simulink library "vhit_control_library"  (R2023a)
settings: Solver=VariableStepAuto  StartTime=0.0  StopTime=10.0  RelTol=1e-3
undefined symbols (not defined in the file): bit, cstElctSpdMaxVal, cstSlowTaskSampTime, parDirCurrMaxVal, parElctSpdMaxVal, parFluxObsFiltCoef, parQdrtCurrMaxVal, parRefSpdFallSlewRate, parRefSpdRisSlewRate, PolePairNum
libraries: lib_conversion x90, lib_square_root x11, lib_dynamic_saturator x9, lib_resettable_unit_delay x2, lib_fault_definiteness x1, lib_angle_mapper x1, lib_cart_to_polar_coor_transformer x1, lib_clarke_transform x1, lib_configurable_parameter x1, lib_current_control_decoupling x1, lib_derating_reference_speed_limiter x1, lib_discrete_time_integrator x1
(part 3 of 3)

== system vhit_control_library/lib_FWReferenceCurrentGenerator_0/vss_ActiveReferenceCurrentStrategy/vss_FieldWeakeningStrategy/sss_CurrentMTPALimitComputation/ias_CurrentMTPALimitAsymmetricMotorCondition ==
  lb_mfPermMagFlux : Inport
  Action Port : ActionPort
  Add1 : Sum  Inputs=+-  OutDataTypeStr=Inherit: Inherit via back propagation
  Add2 : Sum  Inputs=+-  OutDataTypeStr=Inherit: Inherit via back propagation
  Add3 : Sum  OutDataTypeStr=Inherit: Same as first input
  Add4 : Sum  Inputs=+-  OutDataTypeStr=Inherit: Same as first input
  Constant3 : Constant  Value=lb_parQdrtIndc
  Constant4 : Constant  Value=lb_parDirIndc
  Constant5 : Constant  Value=lb_parMaxPhsCurr
  Constant6 : Constant  Value=lb_parMaxPhsCurr
  Data Type Duplicate : DataTypeDuplicate
  Divide1 : Product  Inputs=*/  OutDataTypeStr=Inherit: Inherit via back propagation
  Gain : Gain  Gain=4  OutDataTypeStr=Inherit: Same as input
  Gain1 : Gain  Gain=1/2  OutDataTypeStr=Inherit: Inherit via back propagation
  Square{,1..3} (4 alike) : Math  Operator=square  SignedPower=on  OutDataTypeStr=Inherit: Inherit via back propagation
  lib_SquareRoot_1 : lib_square_root/lib_SquareRoot_0  lb_parLktSize=128  lb_parInpDataType=uint16  lb_parOutpDataType=Inherit: Inherit via back propagation
  lib_SquareRoot_2 : lib_square_root/lib_SquareRoot_0  lb_parLktSize=128  lb_parInpDataType=uint16  lb_parOutpDataType=Inherit: Inherit via back propagation
  lib_s16p29b0_1 : lib_conversion/lib_Conversion_0  lb_parDataType=fixdt(1,16,2^-29,0)  lb_parOutpMaxVal=[]  lb_parOutpMinVal=[]  lb_parSatFlag=off
  lib_s16p7b0_1 : lib_conversion/lib_Conversion_0  lb_parDataType=fixdt(1,16,2^-7,0)  lb_parOutpMaxVal=[]  lb_parOutpMinVal=[]  lb_parSatFlag=off
  lib_u16n0b0_1 : lib_conversion/lib_Conversion_0  lb_parDataType=uint16  lb_parOutpMaxVal=[]  lb_parOutpMinVal=[]  lb_parSatFlag=off
  lib_u16n0b0_2 : lib_conversion/lib_Conversion_0  lb_parDataType=uint16  lb_parOutpMaxVal=[]  lb_parOutpMinVal=[]  lb_parSatFlag=off
  lib_u16n0b0_3 : lib_conversion/lib_Conversion_0  lb_parDataType=uint16  lb_parOutpMaxVal=[]  lb_parOutpMinVal=[]  lb_parSatFlag=off
  lib_u16p2b0_1 : lib_conversion/lib_Conversion_0  lb_parDataType=fixdt(0,16,2^-2,0)  lb_parOutpMaxVal=[]  lb_parOutpMinVal=[]  lb_parSatFlag=off
  lib_u16p4b0_4 : lib_conversion/lib_Conversion_0  lb_parDataType=fixdt(0,16,2^-4,0)  lb_parOutpMaxVal=[]  lb_parOutpMinVal=[]  lb_parSatFlag=off
  lb_iDirCurrMTPALim : Outport
  lb_iQdrtCurrMTPALim : Outport  Port=2
  wires:
  [lb_iDirCurrMTPALim] -> lb_iDirCurrMTPALim/1
  [lb_iQdrtCurrMTPALim] -> lb_iQdrtCurrMTPALim/1
  lb_mfPermMagFlux/1 -> [lb_mfPermMagFlux]
  Square3/1 -> lib_u16n0b0_3/1
  Square2/1 -> lib_u16p4b0_4/1
  lib_u16p4b0_4/1 -> Add4/2
  lib_s16p29b0_1/1 -> Gain/1
  lib_SquareRoot_2/1 -> [lb_iQdrtCurrMTPALim]
  lib_s16p7b0_1/1 -> Data Type Duplicate/1, Add2/1
  Add4/1 -> lib_SquareRoot_2/1
  Divide1/1 -> lib_s16p7b0_1/1, Square/1
  lib_u16p2b0_1/1 -> Add3/2
  Add3/1 -> lib_SquareRoot_1/1
  Constant6/1 -> Square3/1
  Constant5/1 -> Square1/1
  Constant4/1 -> Add1/2
  lib_u16n0b0_3/1 -> Add4/1
  lib_u16n0b0_1/1 -> Add3/1
  [lb_mfPermMagFlux] -> Divide1/1
  Gain1/1 -> lib_u16p2b0_1/1
  Add1/1 -> lib_s16p29b0_1/1
  [lb_iDirCurrMTPALim] -> Square2/1
  Square/1 -> lib_u16n0b0_1/1
  Add2/1 -> [lb_iDirCurrMTPALim]
  Constant3/1 -> Add1/1
  lib_SquareRoot_1/1 -> Data Type Duplicate/2, Add2/2
  lib_u16n0b0_2/1 -> Gain1/1
  Gain/1 -> Divide1/2
  Square1/1 -> lib_u16n0b0_2/1

== system vhit_control_library/lib_FWReferenceCurrentGenerator_0/vss_ActiveReferenceCurrentStrategy/vss_FieldWeakeningStrategy/sss_CurrentMTPALimitComputation/ias_CurrentMTPALimitSymmetricMotorCondition ==
  Action Port : ActionPort
  Constant : Constant  Value=0  OutDataTypeStr=Inherit: Inherit via back propagation
  Constant6 : Constant  Value=lb_parMaxPhsCurr
  Data Type Conversion : DataTypeConversion  SaturateOnIntegerOverflow=off  RndMeth=Floor
  lb_iDirCurrMTPALim : Outport
  lb_iQdrtCurrMTPALim : Outport  Port=2
  wires:
  Data Type Conversion/1 -> lb_iQdrtCurrMTPALim/1
  Constant6/1 -> Data Type Conversion/1
  Constant/1 -> lb_iDirCurrMTPALim/1

== system vhit_control_library/lib_FWReferenceCurrentGenerator_0/vss_ActiveReferenceCurrentStrategy/vss_MaximumTorquePerAmpereStrategy/ias_MTPAControlStrategy/sss_MTPAControlStrategy ==
  lb_tqRefTrq : Inport
  lb_mfPermMagFlux : Inport  Port=2
  Prelookup : PreLookup  BreakpointsData=[10:10:110]  BreakpointsSpecification=Even spacing  BreakpointsNumPoints=lb_parTrqSampNum  BreakpointsFirstPoint=lb_parMTPATrqDataFrstVal  BreakpointsSpacing=lb_parMTPATrqDataStepVal  OutputSelection=Index and fraction as bus  RemoveProtectionInput=on  IndexDataTypeStr=uint16  FractionDataTypeStr=fixdt(0,16,2^-15,0)  RndMeth=Simplest
  Prelookup1 : PreLookup  BreakpointsData=[10:10:110]  BreakpointsSpecification=Even spacing  BreakpointsNumPoints=lb_parTempSampNum  BreakpointsFirstPoint=lb_parMTPAPermMagFluxDataFrstVal  BreakpointsSpacing=lb_parMTPAPermMagFluxDataStepVal  OutputSelection=Index and fraction as bus  RemoveProtectionInput=on  IndexDataTypeStr=uint16  FractionDataTypeStr=fixdt(0,16,2^-15,0)  RndMeth=Simplest
  lib_Conversion_1 : lib_conversion/lib_Conversion_0  lb_parDataType=lb_parOutpDataType  lb_parOutpMaxVal=[]  lb_parOutpMinVal=[]  lb_parSatFlag=off
  lkt_MTPAControlStrategy : Interpolation_n-D  Table=lb_parMTPA2DLktMtrx  ExtrapMethod=Clip  RequireIndexFractionAsBus=on  RemoveProtectionIndex=on  OutDataTypeStr=Inherit: Inherit via back propagation  InternalRulePriority=Speed  RndMeth=Simplest
      settings: InputPortMap=u0,u1
  lb_iMTPARefDirCurr : Outport
  wires:
  lb_tqRefTrq/1 -> [lb_tqRefTrq]
  lb_mfPermMagFlux/1 -> [lb_mfPermMagFlux]
  [lb_tqRefTrq] -> Prelookup/1
  [lb_mfPermMagFlux] -> Prelookup1/1
  Prelookup/1 -> lkt_MTPAControlStrategy/1
  Prelookup1/1 -> lkt_MTPAControlStrategy/2
  lkt_MTPAControlStrategy/1 -> lib_Conversion_1/1
  [lb_iMTPARefDirCurr] -> lb_iMTPARefDirCurr/1
  lib_Conversion_1/1 -> [lb_iMTPARefDirCurr]

== system vhit_control_library/lib_FWReferenceCurrentGenerator_0/vss_ActiveReferenceCurrentStrategy/vss_MaximumTorquePerAmpereStrategy/sss_CurrentMTPALimitComputation/ias_CurrentMTPALimitAsymmetricMotorCondition ==
  lb_mfPermMagFlux : Inport
  Action Port : ActionPort
  Add1 : Sum  Inputs=+-  OutDataTypeStr=Inherit: Inherit via back propagation  RndMeth=Simplest
  Add2 : Sum  Inputs=+-  OutDataTypeStr=Inherit: Inherit via back propagation  RndMeth=Simplest
  Add3 : Sum  RndMeth=Simplest  OutDataTypeStr=Inherit: Same as first input
  Add4 : Sum  Inputs=+-  RndMeth=Simplest  OutDataTypeStr=Inherit: Same as first input
  Constant : Constant  OutDataTypeStr=uint16
  Constant3 : Constant  Value=lb_parQdrtIndc
  Constant4 : Constant  Value=lb_parDirIndc
  Constant5 : Constant  Value=lb_parMaxPhsCurr
  Constant6 : Constant  Value=lb_parMaxPhsCurr
  Data Type Duplicate : DataTypeDuplicate
  Divide2 : Product  Inputs=*/  OutDataTypeStr=Inherit: Inherit via back propagation  RndMeth=Simplest
  Gain : Gain  Gain=4  RndMeth=Simplest  OutDataTypeStr=Inherit: Same as input
  Gain1 : Gain  Gain=1/2  OutDataTypeStr=Inherit: Inherit via back propagation  RndMeth=Simplest
  Product : Product  OutDataTypeStr=Inherit: Inherit via back propagation
  Square{,1..3} (4 alike) : Math  Operator=square  SignedPower=on  OutDataTypeStr=Inherit: Inherit via back propagation  RndMeth=Simplest
  lib_SquareRoot_1 : lib_square_root/lib_SquareRoot_0  lb_parLktSize=1024  lb_parInpDataType=uint16  lb_parOutpDataType=Inherit: Inherit via back propagation
  lib_SquareRoot_2 : lib_square_root/lib_SquareRoot_0  lb_parLktSize=128  lb_parInpDataType=uint16  lb_parOutpDataType=Inherit: Inherit via back propagation
  lib_s16n0b0_4 : lib_conversion/lib_Conversion_0  lb_parDataType=uint32  lb_parOutpMaxVal=[]  lb_parOutpMinVal=[]  lb_parSatFlag=off
  lib_s16p29b0_1 : lib_conversion/lib_Conversion_0  lb_parDataType=fixdt(1,16,2^-29,0)  lb_parOutpMaxVal=[]  lb_parOutpMinVal=[]  lb_parSatFlag=off
  lib_s16p7b0_1 : lib_conversion/lib_Conversion_0  lb_parDataType=fixdt(1,16,2^-7,0)  lb_parOutpMaxVal=[]  lb_parOutpMinVal=[]  lb_parSatFlag=off
  lib_u16n0b0_1 : lib_conversion/lib_Conversion_0  lb_parDataType=uint16  lb_parOutpMaxVal=[]  lb_parOutpMinVal=[]  lb_parSatFlag=off
  lib_u16n0b0_2 : lib_conversion/lib_Conversion_0  lb_parDataType=uint16  lb_parOutpMaxVal=[]  lb_parOutpMinVal=[]  lb_parSatFlag=off
  lib_u16n0b0_3 : lib_conversion/lib_Conversion_0  lb_parDataType=uint16  lb_parOutpMaxVal=[]  lb_parOutpMinVal=[]  lb_parSatFlag=off
  lib_u16p2b0_1 : lib_conversion/lib_Conversion_0  lb_parDataType=fixdt(0,16,2^-2,0)  lb_parOutpMaxVal=[]  lb_parOutpMinVal=[]  lb_parSatFlag=off
  lib_u16p4b0_4 : lib_conversion/lib_Conversion_0  lb_parDataType=fixdt(0,16,2^-4,0)  lb_parOutpMaxVal=[]  lb_parOutpMinVal=[]  lb_parSatFlag=off
  lb_iDirCurrMTPALim : Outport
  lb_iQdrtCurrMTPALim : Outport  Port=2
  wires:
  [lb_iDirCurrMTPALim] -> lb_iDirCurrMTPALim/1
  [lb_iQdrtCurrMTPALim] -> lb_iQdrtCurrMTPALim/1
  lb_mfPermMagFlux/1 -> [lb_mfPermMagFlux]
  Square3/1 -> lib_u16n0b0_3/1
  Square2/1 -> lib_u16p4b0_4/1
  lib_u16p4b0_4/1 -> Add4/2
  lib_s16p29b0_1/1 -> Gain/1
  lib_SquareRoot_2/1 -> [lb_iQdrtCurrMTPALim]
  lib_s16p7b0_1/1 -> Data Type Duplicate/1, Add2/1
  Add4/1 -> lib_SquareRoot_2/1
  Product/1 -> lib_s16p7b0_1/1, Square/1
  lib_u16p2b0_1/1 -> Add3/2
  Add3/1 -> lib_SquareRoot_1/1
  Constant6/1 -> Square3/1
  Constant5/1 -> Square1/1
  Constant4/1 -> Add1/2
  lib_u16n0b0_3/1 -> Add4/1
  lib_u16n0b0_1/1 -> Add3/1
  Gain1/1 -> lib_u16p2b0_1/1
  Add1/1 -> lib_s16p29b0_1/1
  [lb_iDirCurrMTPALim] -> Square2/1
  Square/1 -> lib_u16n0b0_1/1
  Add2/1 -> [lb_iDirCurrMTPALim]
  Constant3/1 -> Add1/1
  lib_SquareRoot_1/1 -> Data Type Duplicate/2, Add2/2
  lib_u16n0b0_2/1 -> Gain1/1
  Square1/1 -> lib_u16n0b0_2/1
  Gain/1 -> Divide2/2
  Constant/1 -> Divide2/1
  [lb_mfPermMagFlux] -> Product/1
  Divide2/1 -> lib_s16n0b0_4/1
  lib_s16n0b0_4/1 -> Product/2

== system vhit_control_library/lib_FWReferenceCurrentGenerator_0/vss_ActiveReferenceCurrentStrategy/vss_MaximumTorquePerAmpereStrategy/sss_CurrentMTPALimitComputation/ias_CurrentMTPALimitSymmetricMotorCondition ==
  Action Port : ActionPort
  Constant : Constant  Value=0  OutDataTypeStr=Inherit: Inherit via back propagation
  Constant6 : Constant  Value=lb_parMaxPhsCurr
  Data Type Conversion : DataTypeConversion  SaturateOnIntegerOverflow=off  RndMeth=Floor
  lb_iDirCurrMTPALim : Outport
  lb_iQdrtCurrMTPALim : Outport  Port=2
  wires:
  Data Type Conversion/1 -> lb_iQdrtCurrMTPALim/1
  Constant6/1 -> Data Type Conversion/1
  Constant/1 -> lb_iDirCurrMTPALim/1

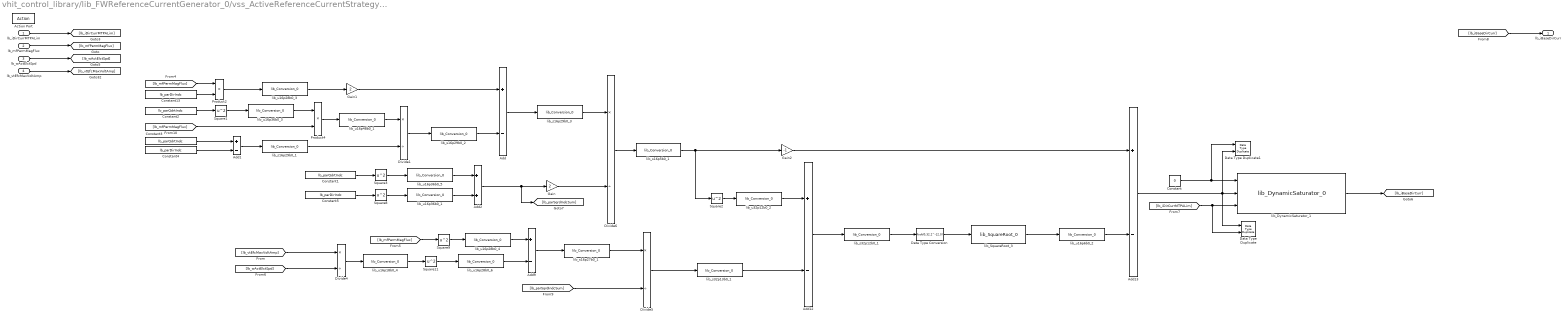
== system vhit_control_library/lib_FWReferenceCurrentGenerator_0/vss_ActiveReferenceCurrentStrategy/vss_FieldWeakeningStrategy/sss_BaseSpeedComputation/ias_CurrentMTPALimitAsymmetricMotorCondition/ias_BaseSpeedExceeded ==
  lb_iDirCurrMTPALim : Inport
  lb_mfPermMagFlux : Inport  Port=2
  lb_wActElctSpd : Inport  Port=3
  lb_vtEfcMaxVoltAmp : Inport  Port=4
  Action Port : ActionPort
  Add{,1,9,12..13} (5 alike) : Sum  Inputs=+-  OutDataTypeStr=Inherit: Inherit via back propagation
  Add2 : Sum  OutDataTypeStr=Inherit: Same as first input
  Constant : Constant  Value=0  OutDataTypeStr=Inherit: Inherit via back propagation
  Constant1 : Constant  Value=lb_parQdrtIndc
  Constant13 : Constant  Value=lb_parDirIndc
  Constant2 : Constant  Value=lb_parQdrtIndc
  Constant3 : Constant  Value=lb_parQdrtIndc
  Constant4 : Constant  Value=lb_parDirIndc
  Constant5 : Constant  Value=lb_parDirIndc
  Data Type Duplicate : DataTypeDuplicate
  Data Type Duplicate1 : DataTypeDuplicate
  Data Type Conversion : DataTypeConversion  OutDataTypeStr=fixdt(0,32,2^-12,0)  SaturateOnIntegerOverflow=off  RndMeth=Floor
  Divide{1,4..6} (4 alike) : Product  Inputs=*/  OutDataTypeStr=Inherit: Inherit via back propagation
  Gain : Gain  Gain=2  OutDataTypeStr=Inherit: Same as input
  Gain1 : Gain  Gain=2  OutDataTypeStr=Inherit: Same as input
  Gain2 : Gain  Gain=-1  OutDataTypeStr=Inherit: Same as input
  Product2 : Product  OutDataTypeStr=Inherit: Inherit via back propagation
  Product4 : Product  OutDataTypeStr=Inherit: Inherit via back propagation
  Square{1,3,8..9,11} (5 alike) : Math  Operator=square  SignedPower=on  OutDataTypeStr=Inherit: Inherit via back propagation
  Square2 : Math  Operator=square  SignedPower=on  OutDataTypeStr=Inherit: Inherit via back propagation  SaturateOnIntegerOverflow=off
  lib_DynamicSaturator_1 : lib_dynamic_saturator/lib_DynamicSaturator_0
  lib_SquareRoot_3 : lib_square_root/lib_SquareRoot_0  lb_parLktSize=128  lb_parInpDataType=uint16  lb_parOutpDataType=Inherit: Inherit via back propagation
  lib_s16p27b0_1 : lib_conversion/lib_Conversion_0  lb_parDataType=fixdt(1,16,2^-27,0)  lb_parOutpMaxVal=[]  lb_parOutpMinVal=[]  lb_parSatFlag=off
  lib_s16p29b0_1 : lib_conversion/lib_Conversion_0  lb_parDataType=fixdt(1,16,2^-29,0)  lb_parOutpMaxVal=[]  lb_parOutpMinVal=[]  lb_parSatFlag=off
  lib_s16p29b0_2 : lib_conversion/lib_Conversion_0  lb_parDataType=fixdt(1,16,2^-29,0)  lb_parOutpMaxVal=[]  lb_parOutpMinVal=[]  lb_parSatFlag=off
  lib_s16p29b0_3 : lib_conversion/lib_Conversion_0  lb_parDataType=fixdt(1,16,2^-29,0)  lb_parOutpMaxVal=[]  lb_parOutpMinVal=[]  lb_parSatFlag=off
  lib_s16p5b0_1 : lib_conversion/lib_Conversion_0  lb_parDataType=fixdt(1,16,2^-5,0)  lb_parOutpMaxVal=[]  lb_parOutpMinVal=[]  lb_parSatFlag=off
  lib_s32p12b0_1 : lib_conversion/lib_Conversion_0  lb_parDataType=fixdt(1,32,2^-12,0)  lb_parOutpMaxVal=[]  lb_parOutpMinVal=[]  lb_parSatFlag=off
  lib_s32p13b0_1 : lib_conversion/lib_Conversion_0  lb_parDataType=fixdt(1,32,2^-12,0)  lb_parOutpMaxVal=[]  lb_parOutpMinVal=[]  lb_parSatFlag=off
  lib_u16p18b0_4 : lib_conversion/lib_Conversion_0  lb_parDataType=fixdt(0,16,2^-18,0)  lb_parOutpMaxVal=[]  lb_parOutpMinVal=[]  lb_parSatFlag=off
  lib_u16p28b0_3 : lib_conversion/lib_Conversion_0  lb_parDataType=fixdt(0,16,2^-28,0)  lb_parOutpMaxVal=[]  lb_parOutpMinVal=[]  lb_parSatFlag=off
  lib_u16p28b0_4 : lib_conversion/lib_Conversion_0  lb_parDataType=fixdt(0,16,2^-28,0)  lb_parOutpMaxVal=[]  lb_parOutpMinVal=[]  lb_parSatFlag=off
  lib_u16p28b0_6 : lib_conversion/lib_Conversion_0  lb_parDataType=fixdt(0,16,2^-28,0)  lb_parOutpMaxVal=[]  lb_parOutpMinVal=[]  lb_parSatFlag=off
  lib_u16p36b0_1 : lib_conversion/lib_Conversion_0  lb_parDataType=fixdt(0,16,2^-36,0)  lb_parOutpMaxVal=[]  lb_parOutpMinVal=[]  lb_parSatFlag=off
  lib_u16p36b0_3 : lib_conversion/lib_Conversion_0  lb_parDataType=fixdt(0,16,2^-36,0)  lb_parOutpMaxVal=[]  lb_parOutpMinVal=[]  lb_parSatFlag=off
  lib_u16p36b0_5 : lib_conversion/lib_Conversion_0  lb_parDataType=fixdt(0,16,2^-36,0)  lb_parOutpMaxVal=[]  lb_parOutpMinVal=[]  lb_parSatFlag=off
  lib_u16p48b0_1 : lib_conversion/lib_Conversion_0  lb_parDataType=fixdt(0,16,2^-48,0)  lb_parOutpMaxVal=[]  lb_parOutpMinVal=[]  lb_parSatFlag=off
  lib_u16p6b0_2 : lib_conversion/lib_Conversion_0  lb_parDataType=fixdt(0,16,2^-6,0)  lb_parOutpMaxVal=[]  lb_parOutpMinVal=[]  lb_parSatFlag=off
  lib_u32p12b0_2 : lib_conversion/lib_Conversion_0  lb_parDataType=fixdt(0,32,2^-12,0)  lb_parOutpMaxVal=[]  lb_parOutpMinVal=[]  lb_parSatFlag=off
  lb_iBaseDirCurr : Outport
  wires:
  [lb_iBaseDirCurr] -> lb_iBaseDirCurr/1
  lb_wActElctSpd/1 -> [lb_wActElctSpd]
  lb_mfPermMagFlux/1 -> [lb_mfPermMagFlux]
  Add13/1 -> lib_DynamicSaturator_1/2, Data Type Duplicate1/2, Data Type Duplicate/1
  lib_s16p29b0_3/1 -> Divide6/1
  lib_u16p6b0_2/1 -> Add13/2
  [lb_iDirCurrMTPALim] -> Data Type Duplicate/2, lib_DynamicSaturator_1/3
  lib_u16p28b0_6/1 -> Add9/2
  lib_s16p29b0_1/1 -> Divide1/2
  Divide5/1 -> lib_s32p13b0_1/1
  lib_s32p13b0_1/1 -> Add12/2
  Constant/1 -> Data Type Duplicate1/1, lib_DynamicSaturator_1/1
  Gain2/1 -> Add13/1
  Square3/1 -> lib_u16p36b0_5/1
  Square8/1 -> lib_u16p36b0_1/1
  lib_u16p36b0_5/1 -> Add2/1
  Square9/1 -> lib_u16p28b0_4/1
  Square1/1 -> lib_u16p36b0_3/1
  [lb_mfPermMagFlux] -> Square9/1
  Product2/1 -> lib_u16p28b0_3/1
  Constant2/1 -> Square1/1
  Divide6/1 -> lib_s16p5b0_1/1
  [lb_wActElctSpd] -> Divide4/2
  lib_u16p28b0_4/1 -> Add9/1
  Gain1/1 -> Add/1
  [lb_vtEfcMaxVoltAmp] -> Divide4/1
  Constant13/1 -> Product2/2
  Gain/1 -> Divide6/2
  Divide4/1 -> lib_u16p18b0_4/1
  Square11/1 -> lib_u16p28b0_6/1
  [lb_mfPermMagFlux] -> Product2/1
  lib_u16p28b0_3/1 -> Gain1/1
  Constant4/1 -> Add1/2
  lib_s32p12b0_1/1 -> Data Type Conversion/1
  Add1/1 -> lib_s16p29b0_1/1
  Constant1/1 -> Square3/1
  lib_s16p29b0_2/1 -> Add/2
  lib_SquareRoot_3/1 -> lib_u16p6b0_2/1
  lib_u32p12b0_2/1 -> Add12/1
  Square2/1 -> lib_u32p12b0_2/1
  lib_u16p36b0_1/1 -> Add2/2
  lib_DynamicSaturator_1/1 -> [lb_iBaseDirCurr]
  [lb_parSqrdIndcSum] -> Divide5/2
  Add12/1 -> lib_s32p12b0_1/1
  Constant5/1 -> Square8/1
  [lb_mfPermMagFlux] -> Product4/2
  lib_s16p27b0_1/1 -> Divide5/1
  Constant3/1 -> Add1/1
  Add/1 -> lib_s16p29b0_3/1
  Product4/1 -> lib_u16p48b0_1/1
  lib_u16p48b0_1/1 -> Divide1/1
  Divide1/1 -> lib_s16p29b0_2/1
  lib_s16p5b0_1/1 -> Gain2/1, Square2/1
  lib_u16p18b0_4/1 -> Square11/1
  Add2/1 -> Gain/1, [lb_parSqrdIndcSum]
  lib_u16p36b0_3/1 -> Product4/1
  Add9/1 -> lib_s16p27b0_1/1
  lb_iDirCurrMTPALim/1 -> [lb_iDirCurrMTPALim]
  Data Type Conversion/1 -> lib_SquareRoot_3/1
  lb_vtEfcMaxVoltAmp/1 -> [lb_vtEfcMaxVoltAmp]

== system vhit_control_library/lib_FWReferenceCurrentGenerator_0/vss_ActiveReferenceCurrentStrategy/vss_FieldWeakeningStrategy/sss_BaseSpeedComputation/ias_CurrentMTPALimitAsymmetricMotorCondition/ias_BaseSpeedLimitExceeded ==
  lb_iDirCurrMTPALim : Inport
  Action Port : ActionPort
  Constant : Constant  Value=0  OutDataTypeStr=Inherit: Inherit via back propagation
  Data Type Duplicate : DataTypeDuplicate
  lb_iBaseDirCurr : Outport
  wires:
  Constant/1 -> Data Type Duplicate/1, lb_iBaseDirCurr/1
  lb_iDirCurrMTPALim/1 -> Data Type Duplicate/2

== system vhit_control_library/lib_FWReferenceCurrentGenerator_0/vss_ActiveReferenceCurrentStrategy/vss_FieldWeakeningStrategy/sss_BaseSpeedComputation/ias_CurrentMTPALimitAsymmetricMotorCondition/ias_BaseSpeedNotExceeded ==
  lb_iDirCurrMTPALim : Inport
  Action Port : ActionPort
  lb_iBaseDirCurr : Outport
  wires:
  lb_iDirCurrMTPALim/1 -> lb_iBaseDirCurr/1

== system vhit_control_library/lib_FWReferenceCurrentGenerator_0/vss_ActiveReferenceCurrentStrategy/vss_FieldWeakeningStrategy/sss_BaseSpeedComputation/ias_CurrentMTPALimitSymmetricMotorCondition/ias_BaseSpeedExceeded ==
  lb_mfPermMagFlux : Inport
  lb_wActElctSpd : Inport  Port=2
  lb_vtEfcMaxVoltAmp : Inport  Port=3
  Action Port : ActionPort
  Add9 : Sum  Inputs=+-  OutDataTypeStr=Inherit: Inherit via back propagation
  Divide4 : Product  Inputs=*/  OutDataTypeStr=Inherit: Inherit via back propagation
  Square11 : Math  Operator=square  SignedPower=on  OutDataTypeStr=Inherit: Inherit via back propagation
  Square9 : Math  Operator=square  SignedPower=on  OutDataTypeStr=Inherit: Inherit via back propagation
  lib_SquareRoot_1 : lib_square_root/lib_SquareRoot_0  lb_parLktSize=128  lb_parInpDataType=uint16  lb_parOutpDataType=Inherit: Inherit via back propagation
  lib_u16n0b0_1 : lib_conversion/lib_Conversion_0  lb_parDataType=uint16  lb_parOutpMaxVal=[]  lb_parOutpMinVal=[]  lb_parSatFlag=off
  lib_u16p18b0_4 : lib_conversion/lib_Conversion_0  lb_parDataType=fixdt(0,16,2^-18,0)  lb_parOutpMaxVal=[]  lb_parOutpMinVal=[]  lb_parSatFlag=off
  lib_u16p28b0_4 : lib_conversion/lib_Conversion_0  lb_parDataType=fixdt(0,16,2^-28,0)  lb_parOutpMaxVal=[]  lb_parOutpMinVal=[]  lb_parSatFlag=off
  lib_u16p28b0_6 : lib_conversion/lib_Conversion_0  lb_parDataType=fixdt(0,16,2^-28,0)  lb_parOutpMaxVal=[]  lb_parOutpMinVal=[]  lb_parSatFlag=off
  lb_iBaseQdrtCurr : Outport
  wires:
  lib_u16n0b0_1/1 -> lib_SquareRoot_1/1
  [lb_wActElctSpd] -> Divide4/2
  Square9/1 -> lib_u16p28b0_4/1
  [lb_mfPermMagFlux] -> Square9/1
  Square11/1 -> lib_u16p28b0_6/1
  Add9/1 -> lib_u16n0b0_1/1
  Divide4/1 -> lib_u16p18b0_4/1
  [lb_vtEfcMaxVoltAmp] -> Divide4/1
  lib_u16p18b0_4/1 -> Square11/1
  lib_SquareRoot_1/1 -> [lb_iBaseQdrtCurr]
  lib_u16p28b0_6/1 -> Add9/1
  lib_u16p28b0_4/1 -> Add9/2
  [lb_iBaseDirCurr] -> lb_iBaseQdrtCurr/1
  lb_wActElctSpd/1 -> [lb_wActElctSpd]
  lb_mfPermMagFlux/1 -> [lb_mfPermMagFlux]
  lb_vtEfcMaxVoltAmp/1 -> [lb_vtEfcMaxVoltAmp]

== system vhit_control_library/lib_FWReferenceCurrentGenerator_0/vss_ActiveReferenceCurrentStrategy/vss_FieldWeakeningStrategy/sss_BaseSpeedComputation/ias_CurrentMTPALimitSymmetricMotorCondition/ias_BaseSpeedLimitExceeded ==
  Action Port : ActionPort
  Constant : Constant  Value=0  OutDataTypeStr=Inherit: Inherit via back propagation
  lb_iBaseQdrtCurr : Outport
  wires:
  Constant/1 -> lb_iBaseQdrtCurr/1

== system vhit_control_library/lib_FWReferenceCurrentGenerator_0/vss_ActiveReferenceCurrentStrategy/vss_FieldWeakeningStrategy/sss_BaseSpeedComputation/ias_CurrentMTPALimitSymmetricMotorCondition/ias_BaseSpeedNotExceeded ==
  lb_iQdrtCurrMTPALim : Inport
  Action Port : ActionPort
  lb_iBaseQdrtCurr : Outport
  wires:
  lb_iQdrtCurrMTPALim/1 -> lb_iBaseQdrtCurr/1

== stateflow chart vhit_control_library/lib_HysDeb_1/sfc_Debounce1 ==
  state Wait
    en:  lb_cntDebCond = uint16(0);
    lb_genOutp = false;
  state Confirming
    /*Set Bit0*/
    en:lb_cntDebCond++;lb_genOutp = false;
    du:lb_cntDebCond++;
  state Confirm
    /*Set Bit0 Bit1*/
    en: lb_cntDebCond = uint16(0);lb_genOutp = true;
  (default) -> (junction 179)
  (junction 179) -> (junction 181) [order 1] : /*There is Fault*/
      | [lb_bolInp]
  (junction 181) -> (junction 184) [order 1] : /*Direct Confirm*/
      | [lb_cntDebConf == uint16(0)]
  (junction 179) -> Wait [order 2]
  (junction 181) -> Confirming [order 2]
  (junction 184) -> Confirm
  Confirming -> Wait [order 1] : /*There is no Fault*/
      | [!lb_bolInp]
  (junction 212) -> Confirming [order 2] : /*Need Debounce*/
  Wait -> (junction 212) : /*There is Fault*/
      | [lb_bolInp]
  (junction 212) -> Confirm [order 1] : /*Direct Confirm*/
      | [lb_cntDebConf == uint16(0)]
  Confirm -> Wait : /*There is no Fault*/
      | [!lb_bolInp]
  Confirming -> Confirm [order 2] : /*Fault Is Confirmed*/
      | [lb_cntDebCond >= lb_cntDebConf]
  data: lb_bolInp input boolean; lb_cntDebConf input uint16; lb_genOutp output boolean; lb_cntDebCond local uint16
  data lb_bolInp settings: description=$TL$ inheritscaling=1; $TL$
  data lb_cntDebConf settings: description=$TL$ inheritscaling=1; $TL$
  data lb_genOutp settings: description=$TL$ type=UInt8; $TL$
  data lb_cntDebCond settings: description=$TL$ type=UInt16; $TL$

== stateflow chart vhit_control_library/lib_RateLimiter_YXQ_0/Chart ==
  (default) -> (junction 26)
  (junction 26) -> (junction 30) [order 1] : [~lb_incrRatLimOn  && lb_decrRatLimOn]
  (junction 26) -> (junction 1) [order 2]
  (junction 30) -> (junction 32) : {lb_noRatLimReq = false;
      | lb_incrRatLimReq = false;
      | lb_decrRatLimReq = true;}
  (junction 1) -> (junction 4) [order 1] : [lb_incrRatLimOn  && ~lb_decrRatLimOn]
  (junction 1) -> (junction 3) [order 2] : {lb_noRatLimReq = true;
      | lb_incrRatLimReq = false;
      | lb_decrRatLimReq = false;}
  (junction 4) -> (junction 6) : {lb_noRatLimReq = false;
      | lb_incrRatLimReq = true;
      | lb_decrRatLimReq = false;}
  (junction 6) -> (junction 3)
  (junction 3) -> (junction 28)
  (junction 32) -> (junction 28)
  (junction 28) -> (junction 38)
  data: lb_incrRatLimOn input boolean; lb_decrRatLimOn input boolean; lb_noRatLimReq output boolean; lb_incrRatLimReq output boolean; lb_decrRatLimReq output boolean

== stateflow chart vhit_control_library/lib_FWReferenceCurrentGenerator_0/vss_ActiveReferenceCurrentStrategy/vss_FieldWeakeningStrategy/sss_MTPAAndFWTransitionLogic/sfc_MTPAAndFWTransitionLogic ==
  state MTPA_status
    en:
    lb_bolFWCond = false;
  state FW_status
    en:
    lb_bolFWCond = true;
  (default) -> MTPA_status
  MTPA_status -> FW_status : [lb_bolBaseSpdExcd && lb_bolBaseDirCurrExcd && ...
      | lb_bolMaxVoltExcd && lb_bolRatSplyVoltCond]
  FW_status -> MTPA_status : [not(lb_bolBaseSpdExcd && lb_bolBaseDirCurrExcd && ...
      | lb_bolMaxVoltExcd && lb_bolRatSplyVoltCond)]
  data: lb_bolBaseSpdExcd input boolean; lb_bolBaseDirCurrExcd input boolean; lb_bolMaxVoltExcd input boolean; lb_bolFWCond output boolean; lb_bolRatSplyVoltCond input boolean

== stateflow chart vhit_control_library/lib_HysDeb_1/sfc_Debounce ==
  state Wait
    en:  lb_cntDebCond = uint16(0);
    lb_genOutp = false;
  state Confirming
    /*Set Bit0*/
    en:lb_cntDebCond++;lb_genOutp = false;
    du:lb_cntDebCond++;
  state Confirm
    /*Set Bit0 Bit1*/
    en: lb_cntDebCond = uint16(0);lb_genOutp = true;
  (default) -> (junction 179)
  (junction 179) -> (junction 181) [order 1] : /*There is Fault*/
      | [lb_bolInp]
  (junction 181) -> (junction 184) [order 1] : /*Direct Confirm*/
      | [lb_cntDebConf == uint16(0)]
  (junction 179) -> Wait [order 2]
  (junction 181) -> Confirming [order 2]
  (junction 184) -> Confirm
  Confirming -> Wait [order 1] : /*There is no Fault*/
      | [!lb_bolInp]
  (junction 212) -> Confirming [order 2] : /*Need Debounce*/
  Wait -> (junction 212) : /*There is Fault*/
      | [lb_bolInp]
  (junction 212) -> Confirm [order 1] : /*Direct Confirm*/
      | [lb_cntDebConf == uint16(0)]
  Confirm -> Wait : /*There is no Fault*/
      | [!lb_bolInp]
  Confirming -> Confirm [order 2] : /*Fault Is Confirmed*/
      | [lb_cntDebCond >= lb_cntDebConf]
  data: lb_bolInp input boolean; lb_cntDebConf input uint16; lb_genOutp output boolean; lb_cntDebCond local uint16
  data lb_bolInp settings: description=$TL$ inheritscaling=1; $TL$
  data lb_cntDebConf settings: description=$TL$ inheritscaling=1; $TL$
  data lb_genOutp settings: description=$TL$ type=UInt8; $TL$
  data lb_cntDebCond settings: description=$TL$ type=UInt16; $TL$
